simulink model "gfm_standalone"  (R2024a)
settings: Solver=VariableStepAuto  StartTime=0  StopTime=5  RelTol=1e-3
values from neighbouring files (symbols this model uses):
  Cf_pu = 0.03    [main__gfm.m]    (also in main_parallel.m; main_parallel_alt.m; main_standalone.m; scr.m)
  Cs_pu = 0.3    [main_parallel.m]    (also in main_parallel_alt.m; main_standalone.m)
  Dp = 0.02    [main__gfm.m]    (also in main_parallel.m; main_parallel_alt.m; main_standalone.m; scr.m)
  Dq = 0.3    [main__gfm.m]    (also in main_parallel.m; main_parallel_alt.m; main_standalone.m; scr.m)
  fac = 0    [main__gfm.m]    (also in main_parallel.m; main_parallel_alt.m; main_standalone.m; scr.m)
  H = 1.2    [main__gfm.m]    (also in main_parallel.m = 0.3; main_parallel_alt.m = 0.3; main_standalone.m; scr.m)
  I_load = Vpcc0/Zload_pu    [main__gfm.m]    (also in main_parallel.m = Vpcc/Zload_pu; main_parallel_alt.m = Vpoc/Zload_pu; main_standalone.m; scr.m)
  Ic = (Vconv-Vlcl)/(Rc_pu+1i*Lc_pu)    [main__gfm.m]    (also in main_standalone.m; scr.m; ss_RX.m; test_droop_gain.m)
  If = (Vlcl - Vload) / Zf_pu    [main_standalone.m]
  Ig = (Vlcl - Vinf) / Z_pu    [main__gfm.m]    (also in main_standalone.m = (Vload - Vinf) / Z_pu; scr.m; ss_RX.m; test_droop_gain.m)
  kfi = 0    [main__gfm.m]    (also in main_parallel.m; main_parallel_alt.m; main_standalone.m; scr.m)
  kii = Rc_pu / L * kpi    [main__gfm.m]    (also in main_parallel.m; main_parallel_alt.m; main_standalone.m; scr.m)
  kiq = 0.1    [main__gfm.m]    (also in main_parallel.m = 0.01; main_parallel_alt.m = 0.01; main_standalone.m; scr.m)
  kivd = 100    [main__gfm.m]    (also in main_parallel.m = 50; main_parallel_alt.m = 50; main_standalone.m; scr.m)
  kivq = 100    [main__gfm.m]    (also in main_parallel.m = 50; main_parallel_alt.m = 50; main_standalone.m; scr.m)
  kpi = 2 * pi * f_bw * L    [main__gfm.m]    (also in main_parallel.m; main_parallel_alt.m; main_standalone.m; scr.m)
  kpvd = 0.1    [main__gfm.m]    (also in main_parallel.m = 0.45; main_parallel_alt.m = 0.45; main_standalone.m; scr.m)
  kpvq = 0.1    [main__gfm.m]    (also in main_parallel.m = 0.45; main_parallel_alt.m = 0.45; main_standalone.m; scr.m = 1)
  Lc_pu = Lc / Lb    [main__gfm.m]    (also in main_parallel.m; main_parallel_alt.m; main_standalone.m; scr.m)
  Lg_pu = 0.5    [main__gfm.m]    (also in main_parallel.m = 0.0166666666667; main_parallel_alt.m = 0.0166666666667; main_standalone.m; scr.m = Lg_pux)
  Lgf_pu = Lgf/Lb    (= 0.0166666666667)    [main_parallel.m]    (also in main_parallel_alt.m; main_standalone.m)
  mu = 0.005    [main__gfm.m]    (also in main_standalone.m; scr.m; ss_RX.m; test_droop_gain.m)
  Pref = -line_flow(3,4)    [main__gfm.m]    (also in main_standalone.m = -line_flow(5,4); scr.m; ss_RX.m; test_droop_gain.m)
  PsiId0 = real(Vconv_c)-real(Vpcc_c)+X*imag(Ipcc_c)    [main__gfm.m]    (also in main_standalone.m; scr.m; ss_RX.m; test_droop_gain.m)
  PsiIq0 = imag(Vconv_c)-imag(Vpcc_c)-X*real(Ipcc_c)    [main__gfm.m]    (also in main_standalone.m; scr.m; ss_RX.m; test_droop_gain.m)
  PsiP0 = real(Ipcc_c)-wCpu*imag(Vpcc_c)*fac+imag(Ipcc_c)*kfi    [main__gfm.m]    (also in main_standalone.m; scr.m; ss_RX.m; test_droop_gain.m)
  PsiV0 = imag(Ipcc_c)+wCpu*real(Vpcc_c)*fac+real(Ipcc_c)*kfi    [main__gfm.m]    (also in main_standalone.m; scr.m; ss_RX.m; test_droop_gain.m)
  Qref = -line_flow(3,5)    [main__gfm.m]    (also in main_standalone.m = -line_flow(5,5); scr.m; ss_RX.m; test_droop_gain.m)
  Rc_pu = Rc / Zb    (= 5.19390581717e-06)    [main__gfm.m]    (also in main_parallel.m; main_parallel_alt.m; main_standalone.m; scr.m)
  Rf_pu = Rf / Zb    [main__gfm.m]    (also in main_parallel.m; main_parallel_alt.m; main_standalone.m; scr.m)
  Rg_pu = XrXg*Lg_pu    (= 0)    [main__gfm.m]    (also in main_standalone.m; scr.m; ss_RX.m; test_droop_gain.m)
  Rs_pu = 0.1    [main_parallel.m]    (also in main_parallel_alt.m; main_standalone.m)
  Vcf0 = Vlcl+Rf_pu*Icf    [main__gfm.m]    (also in main_standalone.m; scr.m; ss_RX.m; test_droop_gain.m)
  Vconv_c = Vconv * exp(-1i*theta_ref)    [main__gfm.m]    (also in main_standalone.m; scr.m; ss_RX.m; test_droop_gain.m)
  Vinf = V0(3,1)    [main__gfm.m]    (also in main_parallel.m = V0(6,1); main_parallel_alt.m = V0(6,1); main_standalone.m = V0(4,1); scr.m)
  Vpcc0 = Vlcl    [main__gfm.m]    (also in main_standalone.m = Vload; scr.m; ss_RX.m; test_droop_gain.m)
  Vs = Vpcc + Rs_pu*Igf    [main_parallel.m]    (also in main_parallel_alt.m = Vpoc + Rs_pu*Igf; main_standalone.m = Vload+Rs_pu*Ibf)
  wCpu = Zb * wb * Cf    (= 0.03)    [main__gfm.m]    (also in main_parallel.m; main_parallel_alt.m; main_standalone.m; scr.m)
  wLpu = X    [main__gfm.m]    (also in main_parallel.m; main_parallel_alt.m; main_standalone.m; scr.m)
  Zload_pu = inv(YL(2,2))    [main__gfm.m]    (also in main_parallel.m = inv(YL(3,3)); main_parallel_alt.m = inv(YL(3,3)); main_standalone.m = inv(YL(3,3)); scr.m)
settings Model: Creator=HP  LastModifiedBy=HP
settings DataIOCC: SaveFormat=StructureWithTime
settings OptimizationCC: BlockReduction=off  BufferReuse=off
settings DebuggingCC: AlgebraicLoopMsg=none

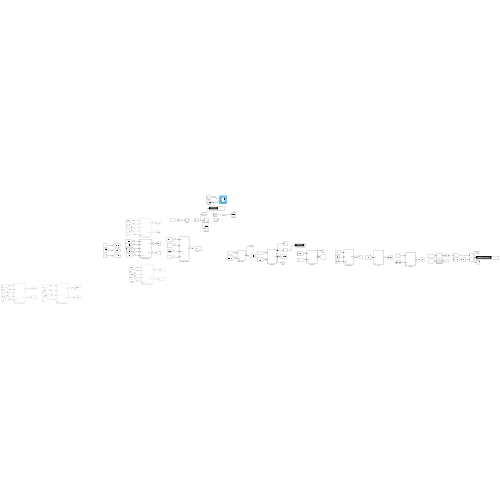
[thumbnail: Simulink's stored preview of the top-level diagram]
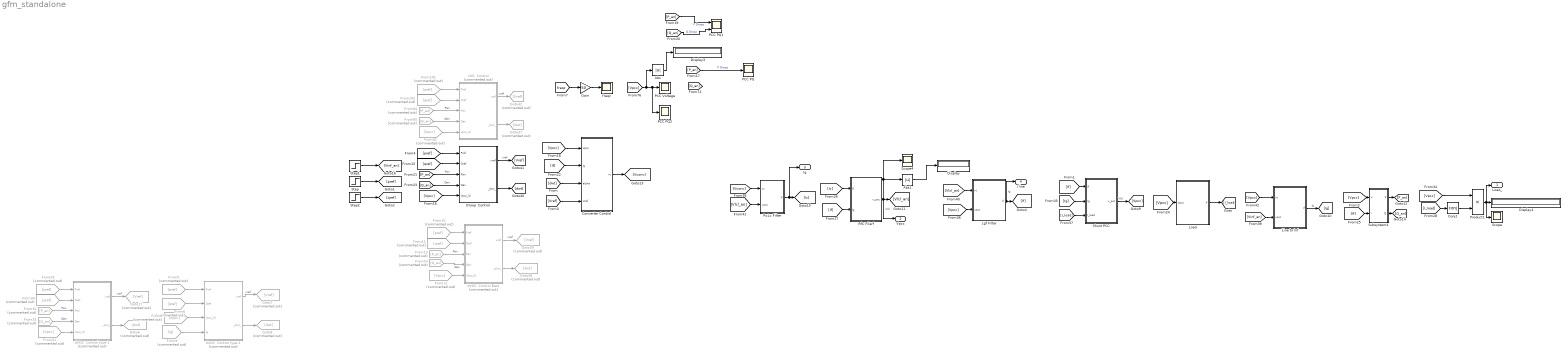
== system gfm_standalone ==
  Abs : Abs  SaturateOnIntegerOverflow=off
  Abs1 : Abs  SaturateOnIntegerOverflow=off
  Conj2 : Math  Operator=conj
  Converter Control : Subsystem
  Display : Display
  Display3 : Display
  Display4 : Display
  Droop  Control : Subsystem  mask{md=Dp, nd=Dq, kiq=0, vref_=Vpcc0}
      mask prompts: md "P droop gain"; nd "Q droop gain"; kiq "KiQ-V"; vref_ "Voltage ref"
      mask DialogControl DescGroupVar Prompt: Outer Control
      mask DialogControl DescTextVar Prompt: Droop Control Block by HIP
  From{5,10,29,101} (4 alike) : From  Commented=on  GotoTag=pref
  From{6,11,30,102} (4 alike) : From  Commented=on  GotoTag=qref
  From{8,12,31,92} (4 alike) : From  Commented=on  GotoTag=Vpcc
  From13 : From  Commented=on  GotoTag=P_an
  From14 : From  Commented=on  GotoTag=Q_an
  From32 : From  Commented=on  GotoTag=P_an
  From33 : From  Commented=on  GotoTag=Q_an
  From9 : From  Commented=on  GotoTag=Ig
  From94 : From  Commented=on  GotoTag=P_an
  From95 : From  Commented=on  GotoTag=Q_an
  Gain : Gain  Gain=50
  Goto{7,17,39,42} (4 alike) : Goto  Commented=on  GotoTag=Vref
  Goto{6,8,37..38} (4 alike) : Goto  Commented=on  GotoTag=dwt
  Lgf Filter : Subsystem  mask{i0=If, R=0, L=Lgf_pu}
      mask prompts: i0 "I initial condition (pu)"; R "R (pu)"; L "L (pu)"
  Line to Inf : Subsystem  mask{i0=Ig, R=Rg_pu, L=Lg_pu}
      mask prompts: i0 "I initial condition (pu)"; R "R (pu)"; L "L (pu)"
  Load : Subsystem  mask{i0=I_load, R=real(Zload_pu), L=imag(Zload_pu)}
      mask prompts: i0 "I initial condition (pu)"; R "R (pu)"; L "L (pu)"
  PCC PQ : Scope
  PCC PQ1 : Scope  NumInputPorts=2
  PCC PQ2 : Scope
  PCC Voltage : Scope
  Product1 : Product
  RcLc Filter : Subsystem  mask{i0=Ic, R=Rc_pu, L=Lc_pu}
      mask prompts: i0 "I initial condition (pu)"; R "R (pu)"; L "L (pu)"
  RfC Filerf : Subsystem  mask{vc0=Vcf0, R=Rf_pu, C=Cf_pu}
      mask prompts: vc0 "initial value Vpcc  (p.u.)"; R "R (pu)"; C "C (pu)"
  Scope : Scope
  Scope4 : Scope
  Shunt PCC : Subsystem  mask{vc0=Vs, R=Rs_pu, C=Cs_pu}
      mask prompts: vc0 "initial value Vpcc  (p.u.)"; R "R (pu)"; C "C (pu)"
  Step : Step  Before=Pref  SampleTime=0
  Step1 : Step  Time=2  Before=Vinf  After=Vinf  SampleTime=0
  Step2 : Step  Before=Qref  After=0.2  SampleTime=0
  Subsystem4 : Subsystem
  VSG  Control : Subsystem  Commented=on  mask{Dp=50, H=H, nd=Dq, kiq=kiq, vref_=Vpcc0}
      mask prompts: Dp "Dp (damping factor)"; H "Inertia Constant"; nd "VSG Q gain"; kiq "KiQ-V"; vref_ "Voltage ref"
      mask DialogControl DescGroupVar Prompt: Outer Control
      mask DialogControl DescTextVar Prompt: VSG Control Block by HIP
  dVOC  Control Best : Subsystem  Commented=on  mask{md=Dp, nd=Dq, mu=mu, vref_=Vpcc0}
      mask prompts: md "P droop gain"; nd "Q droop gain"; mu "mu (V)"; vref_ "Voltage ref"
      mask DialogControl DescGroupVar Prompt: Outer Control
      mask DialogControl DescTextVar Prompt: dVOC Control Block by HIP
  dVOC  Control type 1 : Subsystem  Commented=on  mask{md=Dp, nd=Dq, mu=mu, vref_=Vpcc0}
      mask prompts: md "P droop gain"; nd "Q droop gain"; mu "mu (V)"; vref_ "Voltage ref"
      mask DialogControl DescGroupVar Prompt: Outer Control
      mask DialogControl DescTextVar Prompt: dVOC Control Block by HIP
  dVOC  Control type 2 : Subsystem  Commented=on  mask{md=Dp, nd=Dq, mu=mu, vref_=Vpcc0}
      mask prompts: md "P droop gain"; nd "Q droop gain"; mu "mu (V)"; vref_ "Voltage ref"
      mask DialogControl DescGroupVar Prompt: Outer Control
      mask DialogControl DescTextVar Prompt: dVOC Control Block by HIP
  freqz : Scope
  Load_ : Outport
  Vpcc : Outport  Port=2
  Ig : Outport  Port=3
  I line : Outport  Port=4
  wires:
  [If] -> Converter Control/2(Ig)
  [Vref] -> Converter Control/4(Vref)
  [Vpcc] -> Converter Control/1(Vpcc)
  Converter Control/1(vt) -> [Vconv]
  [dwt] -> Converter Control/3(alpha)
  Step/1 -> [pref]
  Step1/1 -> [Vinf_an]
  Step2/1 -> [qref]
  Gain/1 -> freqz/1
  [freqz] -> Gain/1
  [Vpcc] -> Abs/1, PCC PQ2/1, PCC Voltage/1
  Droop  Control/1(vref) -> [Vref]  "vref"
  From92/1 -> VSG  Control/5(Vpcc_lcl)
  From95/1 -> VSG  Control/4(Qan)  "Qan"
  VSG  Control/2(_dwt_) -> Goto37/1
  Droop  Control/2(_dwt_) -> [dwt]
  From102/1 -> VSG  Control/2(Qref)
  From101/1 -> VSG  Control/1(Pref)
  From94/1 -> VSG  Control/3(Pan)  "Pan"
  VSG  Control/1(vref) -> Goto42/1  "vref"
  [pref] -> Droop  Control/1(Pref)
  [qref] -> Droop  Control/2(Qref)
  [Q_an] -> Droop  Control/4(Qan)  "Qan"
  [P_an] -> Droop  Control/3(Pan)  "Pan"
  [Vpcc] -> Droop  Control/5(Vpcc_lcl)
  [P_an] -> PCC PQ/1  "P Droop"
  dVOC  Control type 1/1(vref) -> Goto17/1  "vref"
  From30/1 -> dVOC  Control type 1/2(Qref)
  dVOC  Control type 1/2(_dwt_) -> Goto6/1
  From29/1 -> dVOC  Control type 1/1(Pref)
  From33/1 -> dVOC  Control type 1/4(Qan)  "Qan"
  From32/1 -> dVOC  Control type 1/3(Pan)  "Pan"
  From31/1 -> dVOC  Control type 1/5(Vpcc_lcl)
  From8/1 -> dVOC  Control type 2/3(Vpcc_lcl)
  From5/1 -> dVOC  Control type 2/1(Pref)
  From6/1 -> dVOC  Control type 2/2(Qref)
  dVOC  Control type 2/2(_dwt_) -> Goto8/1
  dVOC  Control type 2/1(vref) -> Goto7/1  "vref"
  From9/1 -> dVOC  Control type 2/4(Ig)
  Abs/1 -> Display3/1
  dVOC  Control Best/1(vref) -> Goto39/1  "vref"
  dVOC  Control Best/2(_dwt_) -> Goto38/1
  From10/1 -> dVOC  Control Best/1(Pref)
  From11/1 -> dVOC  Control Best/2(Qref)
  From13/1 -> dVOC  Control Best/3(Pan)  "Pan"
  From14/1 -> dVOC  Control Best/4(Qan)  "Qan"
  From12/1 -> dVOC  Control Best/5(Vpcc_lcl)
  [Q_an] -> PCC PQ1/2  "Q Droop"
  [P_an] -> PCC PQ1/1  "P Droop"
  [Vinf_an] -> Line to Inf/2("vpcc ")
  [If] -> RfC Filerf/2("Ig ")
  RcLc Filter/1(if) -> Ig/1, [Ic]
  [Vconv] -> RcLc Filter/1("vt ")
  Lgf Filter/1(if) -> I line/1, [If]  "Ig"
  [Vpcc] -> Subsystem4/1(V)
  [Vpcc] -> Line to Inf/1("vt ")
  [Vlcl_an] -> Lgf Filter/1("vt ")
  [If] -> Subsystem4/2(I)
  Conj2/1 -> Product1/2
  RfC Filerf/1(v_pcc) -> Vpcc/1, Abs1/1, Scope4/1, [Vlcl_an]  "Vlcl"
  Product1/1 -> Load_/1, Scope/1, Display4/1
  [Ic] -> RfC Filerf/1("If ")
  Line to Inf/1(if) -> [Ig]  "Ig"
  [If] -> Shunt PCC/1("If ")
  [I_load] -> Shunt PCC/3(I_load)
  [I_load] -> Conj2/1
  [Ig] -> Shunt PCC/2("Ig ")
  Subsystem4/1(P) -> [P_an]
  [Vpcc] -> Load/1("Vpcc ")
  [Vpcc] -> Lgf Filter/2("vpcc ")
  [Vlcl_an] -> RcLc Filter/2("vpcc ")
  [Vpcc] -> Product1/1
  Abs1/1 -> Display/1
  Subsystem4/2(Q) -> [Q_an]
  Load/1(if) -> [I_load]
  Shunt PCC/1(v_pcc) -> [Vpcc]  "Vlcl"

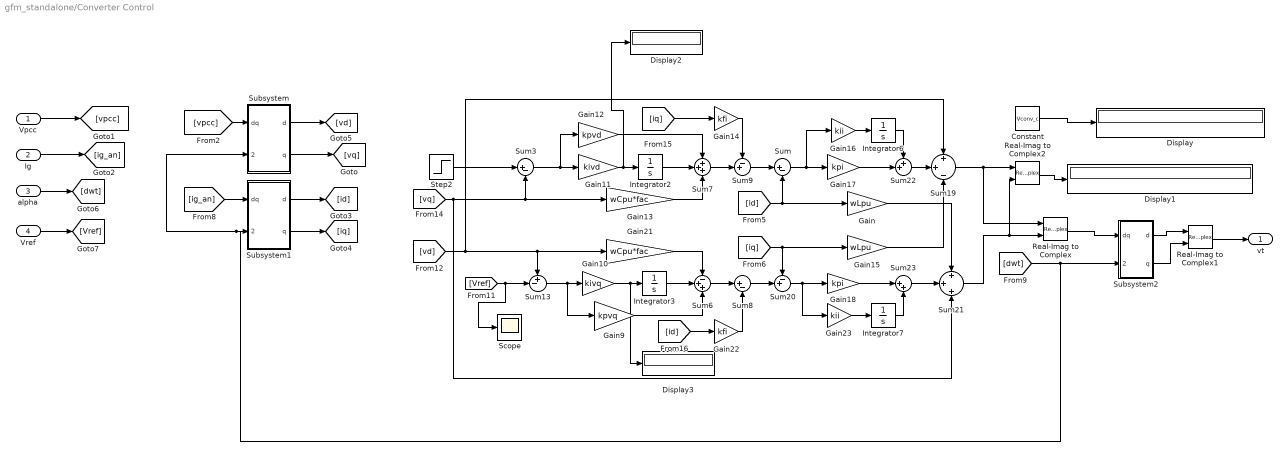
== system gfm_standalone/Converter Control ==
  Vpcc : Inport
  Ig : Inport  Port=2
  alpha : Inport  Port=3
  Vref : Inport  Port=4
  Constant : Constant  Value=Vconv_c
  Display{,1..3} (4 alike) : Display
  Gain : Gain  Gain=wLpu
  Gain10 : Gain  Gain=kivq
  Gain11 : Gain  Gain=kivd
  Gain12 : Gain  Gain=kpvd
  Gain13 : Gain  Gain=wCpu*fac
  Gain14 : Gain  Gain=kfi
  Gain15 : Gain  Gain=wLpu
  Gain16 : Gain  Gain=kii
  Gain17 : Gain  Gain=kpi
  Gain18 : Gain  Gain=kpi
  Gain21 : Gain  Gain=wCpu*fac
  Gain22 : Gain  Gain=kfi
  Gain23 : Gain  Gain=kii
  Gain9 : Gain  Gain=kpvq
  Integrator2 : Integrator  InitialCondition=PsiP0  ContinuousStateAttributes='psi_alpha'
  Integrator3 : Integrator  InitialCondition=PsiV0  ContinuousStateAttributes='psiV'
  Integrator6 : Integrator  InitialCondition=PsiId0  ContinuousStateAttributes='psi_id'
  Integrator7 : Integrator  InitialCondition=PsiIq0  ContinuousStateAttributes='psi_iq'
  Real-Imag to Complex : RealImagToComplex
  Real-Imag to Complex1 : RealImagToComplex
  Real-Imag to Complex2 : RealImagToComplex
  Scope : Scope
  Step2 : Step  After=0  SampleTime=0
  Subsystem : Subsystem
  Subsystem1 : Subsystem
  Subsystem2 : Subsystem
  Sum : Sum  Inputs=|+-
  Sum13 : Sum  Inputs=+-|
  Sum19 : Sum  Inputs=+|+|-
  Sum20 : Sum  Inputs=-+|
  Sum21 : Sum  Inputs=+|+|+
  Sum22 : Sum  Inputs=++|
  Sum23 : Sum  Inputs=|++
  Sum3 : Sum  Inputs=|+-
  Sum6 : Sum  Inputs=-++
  Sum7 : Sum  Inputs=+++
  Sum8 : Sum  Inputs=|+-
  Sum9 : Sum  Inputs=-+|
  vt : Outport
  wires:
  Integrator3/1 -> Sum6/2
  Gain11/1 -> Display2/1, Integrator2/1
  Subsystem/2(q) -> [vq]
  Sum13/1 -> Gain10/1, Gain9/1
  Ig/1 -> [ig_an]
  [vpcc] -> Subsystem/1(dq)
  Subsystem2/2(q) -> Real-Imag to Complex1/2
  Subsystem2/1(d) -> Real-Imag to Complex1/1
  Real-Imag to Complex/1 -> Subsystem2/1(dq)
  [id] -> Sum/2, Gain/1
  Subsystem1/1(d) -> [id]
  [iq] -> Gain15/1, Sum20/1
  Sum21/1 -> Real-Imag to Complex2/2, Real-Imag to Complex/2
  Integrator6/1 -> Sum22/1
  Sum20/1 -> Gain23/1, Gain18/1
  Gain23/1 -> Integrator7/1
  Gain18/1 -> Sum23/1
  Sum22/1 -> Sum19/2
  Gain22/1 -> Sum8/2
  Gain10/1 -> Display3/1, Integrator3/1
  Gain14/1 -> Sum9/1
  Sum8/1 -> Sum20/2
  Sum7/1 -> Sum9/2
  [ig_an] -> Subsystem1/1(dq)
  Gain13/1 -> Sum7/3
  Sum19/1 -> Real-Imag to Complex/1, Real-Imag to Complex2/1
  Sum3/1 -> Gain12/1, Gain11/1
  Gain16/1 -> Integrator6/1
  Sum/1 -> Gain16/1, Gain17/1
  Gain/1 -> Sum21/1
  [Vref] -> Scope/1, Sum13/2
  Gain9/1 -> Sum6/3
  Gain21/1 -> Sum6/1
  Subsystem1/2(q) -> [iq]
  Integrator7/1 -> Sum23/2
  Sum23/1 -> Sum21/2
  Subsystem/1(d) -> [vd]
  [vq] -> Sum3/2, Gain13/1, Sum21/3
  Gain15/1 -> Sum19/3
  [vd] -> Gain21/1, Sum13/1, Sum19/1
  Gain17/1 -> Sum22/2
  [id] -> Gain22/1
  [iq] -> Gain14/1
  Vpcc/1 -> [vpcc]
  Gain12/1 -> Sum7/1
  Sum6/1 -> Sum8/1
  Integrator2/1 -> Sum7/2
  Real-Imag to Complex1/1 -> vt/1
  Sum9/1 -> Sum/1
  [dwt] -> Subsystem1/2(delta_wt), Subsystem/2(delta_wt), Subsystem2/2(d_wt)
  Step2/1 -> Sum3/1
  alpha/1 -> [dwt]
  Vref/1 -> [Vref]
  Constant/1 -> Display/1
  Real-Imag to Complex2/1 -> Display1/1

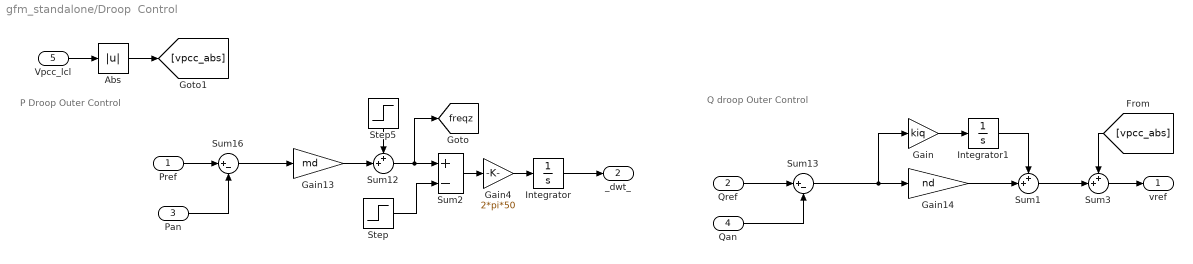
== system gfm_standalone/Droop  Control ==
  note: Q droop Outer Control
  note: P Droop Outer Control
  Pref : Inport
  Qref : Inport  Port=2
  Pan : Inport  Port=3
  Qan : Inport  Port=4
  Vpcc_lcl : Inport  Port=5
  Abs : Abs  SaturateOnIntegerOverflow=off
  Gain : Gain  Gain=kiq
  Gain13 : Gain  Gain=md
  Gain14 : Gain  Gain=nd
  Gain4 : Gain  Gain=2*pi*50
  Integrator : Integrator  InitialCondition=angle(vref_)  ContinuousStateAttributes='theta0'
  Integrator1 : Integrator
  Step : Step  Before=1.00  After=1.000  SampleTime=0
  Step5 : Step  Time=2  Before=1  SampleTime=0
  Sum1 : Sum  Inputs=++|
  Sum12 : Sum  Inputs=++|
  Sum13 : Sum  Inputs=|+-
  Sum16 : Sum  Inputs=|+-
  Sum2 : Sum  Inputs=+-
  Sum3 : Sum  Inputs=++|
  vref : Outport
  _dwt_ : Outport  Port=2
  tag scope: freqz=global
  wires:
  Gain13/1 -> Sum12/2
  Qref/1 -> Sum13/1
  Sum3/1 -> vref/1
  Qan/1 -> Sum13/2
  Pref/1 -> Sum16/1
  Pan/1 -> Sum16/2
  Sum13/1 -> Gain/1, Gain14/1
  Sum2/1 -> Gain4/1
  Gain4/1 -> Integrator/1
  Sum12/1 -> Sum2/1, [freqz]
  Integrator/1 -> _dwt_/1
  Sum16/1 -> Gain13/1
  Step5/1 -> Sum12/1
  Step/1 -> Sum2/2
  Gain/1 -> Integrator1/1
  Gain14/1 -> Sum1/2
  Integrator1/1 -> Sum1/1
  Sum1/1 -> Sum3/2
  Vpcc_lcl/1 -> Abs/1
  Abs/1 -> [vpcc_abs]
  [vpcc_abs] -> Sum3/1

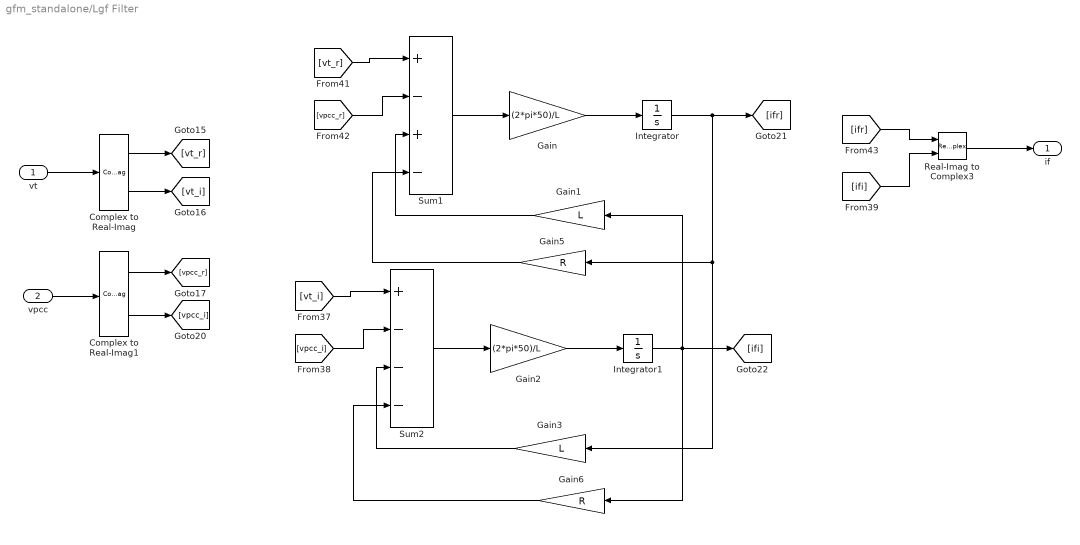
== system gfm_standalone/Lgf Filter ==
  "vt " : Inport
  "vpcc " : Inport  Port=2
  Complex to Real-Imag : ComplexToRealImag
  Complex to Real-Imag1 : ComplexToRealImag
  Gain : Gain  Gain=(2*pi*50)/L
  Gain1 : Gain  Gain=L
  Gain2 : Gain  Gain=(2*pi*50)/L
  Gain3 : Gain  Gain=L
  Gain5 : Gain  Gain=R
  Gain6 : Gain  Gain=R
  Integrator : Integrator  InitialCondition=real(i0)  ContinuousStateAttributes='iline1_re'
  Integrator1 : Integrator  InitialCondition=imag(i0)  ContinuousStateAttributes='iline1_im'
  Real-Imag to Complex3 : RealImagToComplex
  Sum1 : Sum  Inputs=+-+-
  Sum2 : Sum  Inputs=+---
  if : Outport
  wires:
  "vpcc "/1 -> Complex to Real-Imag1/1
  Gain5/1 -> Sum1/4
  Real-Imag to Complex3/1 -> if/1
  Integrator1/1 -> Gain6/1, Gain1/1, [ifi]
  [ifr] -> Real-Imag to Complex3/1
  "vt "/1 -> Complex to Real-Imag/1
  Integrator/1 -> Gain5/1, Gain3/1, [ifr]
  [ifi] -> Real-Imag to Complex3/2
  [vpcc_r] -> Sum1/2
  Gain6/1 -> Sum2/4
  Complex to Real-Imag/1 -> [vt_r]
  Gain1/1 -> Sum1/3
  Complex to Real-Imag/2 -> [vt_i]
  Complex to Real-Imag1/1 -> [vpcc_r]
  Sum2/1 -> Gain2/1
  Gain2/1 -> Integrator1/1
  [vt_i] -> Sum2/1
  [vpcc_i] -> Sum2/2
  [vt_r] -> Sum1/1
  Gain3/1 -> Sum2/3
  Complex to Real-Imag1/2 -> [vpcc_i]
  Gain/1 -> Integrator/1
  Sum1/1 -> Gain/1

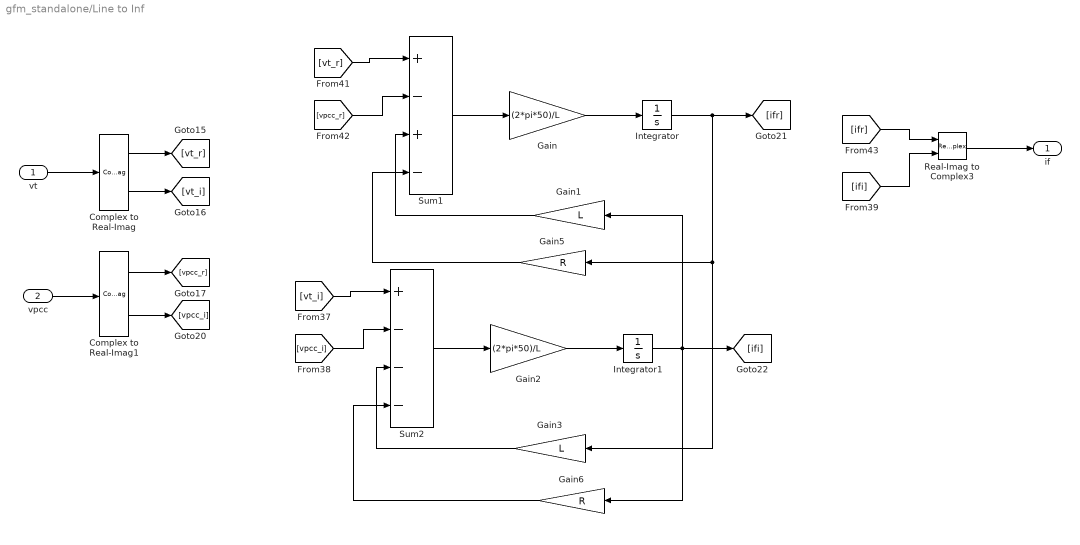
== system gfm_standalone/Line to Inf ==
  "vt " : Inport
  "vpcc " : Inport  Port=2
  Complex to Real-Imag : ComplexToRealImag
  Complex to Real-Imag1 : ComplexToRealImag
  Gain : Gain  Gain=(2*pi*50)/L
  Gain1 : Gain  Gain=L
  Gain2 : Gain  Gain=(2*pi*50)/L
  Gain3 : Gain  Gain=L
  Gain5 : Gain  Gain=R
  Gain6 : Gain  Gain=R
  Integrator : Integrator  InitialCondition=real(i0)  ContinuousStateAttributes='iline1_re'
  Integrator1 : Integrator  InitialCondition=imag(i0)  ContinuousStateAttributes='iline1_im'
  Real-Imag to Complex3 : RealImagToComplex
  Sum1 : Sum  Inputs=+-+-
  Sum2 : Sum  Inputs=+---
  if : Outport
  wires:
  "vpcc "/1 -> Complex to Real-Imag1/1
  Gain5/1 -> Sum1/4
  Real-Imag to Complex3/1 -> if/1
  Integrator1/1 -> Gain6/1, Gain1/1, [ifi]
  [ifr] -> Real-Imag to Complex3/1
  "vt "/1 -> Complex to Real-Imag/1
  Integrator/1 -> Gain5/1, Gain3/1, [ifr]
  [ifi] -> Real-Imag to Complex3/2
  [vpcc_r] -> Sum1/2
  Gain6/1 -> Sum2/4
  Complex to Real-Imag/1 -> [vt_r]
  Gain1/1 -> Sum1/3
  Complex to Real-Imag/2 -> [vt_i]
  Complex to Real-Imag1/1 -> [vpcc_r]
  Sum2/1 -> Gain2/1
  Gain2/1 -> Integrator1/1
  [vt_i] -> Sum2/1
  [vpcc_i] -> Sum2/2
  [vt_r] -> Sum1/1
  Gain3/1 -> Sum2/3
  Complex to Real-Imag1/2 -> [vpcc_i]
  Gain/1 -> Integrator/1
  Sum1/1 -> Gain/1

== system gfm_standalone/Load ==
  "Vpcc " : Inport
  Complex to Real-Imag : ComplexToRealImag
  Gain : Gain  Gain=(2*pi*50)/L
  Gain1 : Gain  Gain=L
  Gain2 : Gain  Gain=(2*pi*50)/L
  Gain3 : Gain  Gain=L
  Gain5 : Gain  Gain=R
  Gain6 : Gain  Gain=R
  Integrator : Integrator  InitialCondition=real(i0)  ContinuousStateAttributes='iload_re'
  Integrator1 : Integrator  InitialCondition=imag(i0)  ContinuousStateAttributes='iload_im'
  Real-Imag to Complex3 : RealImagToComplex
  Sum1 : Sum  Inputs=+-+-
  Sum2 : Sum  Inputs=+---
  if : Outport
  wires:
  Gain5/1 -> Sum1/4
  Real-Imag to Complex3/1 -> if/1
  Integrator1/1 -> Gain6/1, Gain1/1, [ifi]
  [ifr] -> Real-Imag to Complex3/1
  "Vpcc "/1 -> Complex to Real-Imag/1
  Integrator/1 -> Gain5/1, Gain3/1, [ifr]
  [ifi] -> Real-Imag to Complex3/2
  Gain6/1 -> Sum2/4
  Complex to Real-Imag/1 -> [vt_r]
  Gain1/1 -> Sum1/3
  Complex to Real-Imag/2 -> [vt_i]
  Sum2/1 -> Gain2/1
  Gain2/1 -> Integrator1/1
  [vt_i] -> Sum2/1
  [vt_r] -> Sum1/1
  Gain3/1 -> Sum2/3
  Gain/1 -> Integrator/1
  Sum1/1 -> Gain/1

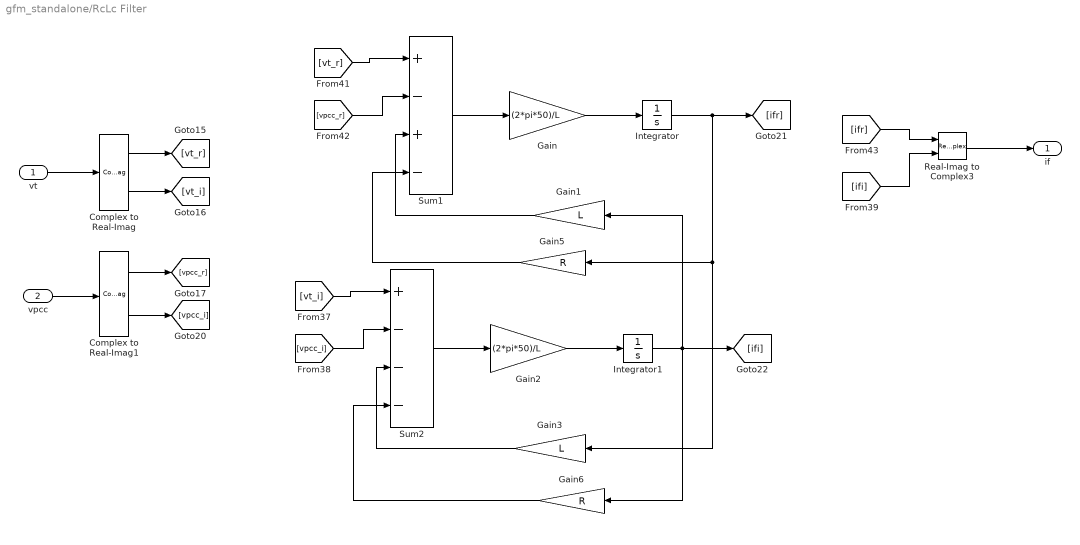
== system gfm_standalone/RcLc Filter ==
  "vt " : Inport
  "vpcc " : Inport  Port=2
  Complex to Real-Imag : ComplexToRealImag
  Complex to Real-Imag1 : ComplexToRealImag
  Gain : Gain  Gain=(2*pi*50)/L
  Gain1 : Gain  Gain=L
  Gain2 : Gain  Gain=(2*pi*50)/L
  Gain3 : Gain  Gain=L
  Gain5 : Gain  Gain=R
  Gain6 : Gain  Gain=R
  Integrator : Integrator  InitialCondition=real(i0)  ContinuousStateAttributes='ig_re'
  Integrator1 : Integrator  InitialCondition=imag(i0)  ContinuousStateAttributes='ig_im'
  Real-Imag to Complex3 : RealImagToComplex
  Sum1 : Sum  Inputs=+-+-
  Sum2 : Sum  Inputs=+---
  if : Outport
  wires:
  "vpcc "/1 -> Complex to Real-Imag1/1
  Gain5/1 -> Sum1/4
  Real-Imag to Complex3/1 -> if/1
  Integrator1/1 -> Gain6/1, Gain1/1, [ifi]
  [ifr] -> Real-Imag to Complex3/1
  "vt "/1 -> Complex to Real-Imag/1
  Integrator/1 -> Gain5/1, Gain3/1, [ifr]
  [ifi] -> Real-Imag to Complex3/2
  [vpcc_r] -> Sum1/2
  Gain6/1 -> Sum2/4
  Complex to Real-Imag/1 -> [vt_r]
  Gain1/1 -> Sum1/3
  Complex to Real-Imag/2 -> [vt_i]
  Complex to Real-Imag1/1 -> [vpcc_r]
  Sum2/1 -> Gain2/1
  Gain2/1 -> Integrator1/1
  [vt_i] -> Sum2/1
  [vpcc_i] -> Sum2/2
  [vt_r] -> Sum1/1
  Gain3/1 -> Sum2/3
  Complex to Real-Imag1/2 -> [vpcc_i]
  Gain/1 -> Integrator/1
  Sum1/1 -> Gain/1

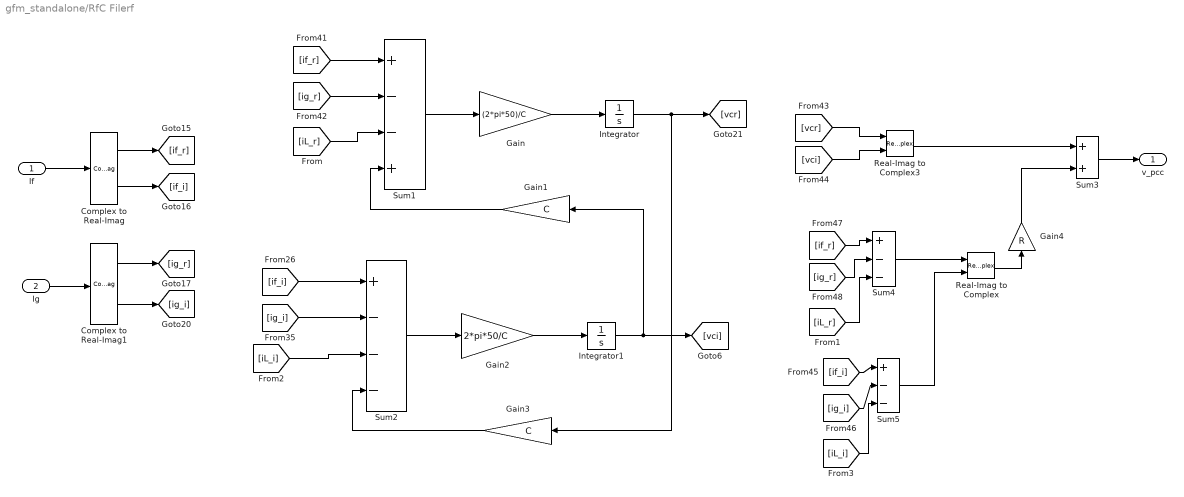
== system gfm_standalone/RfC Filerf ==
  "If " : Inport
  "Ig " : Inport  Port=2
  Complex to Real-Imag : ComplexToRealImag
  Complex to Real-Imag1 : ComplexToRealImag
  Gain : Gain  Gain=(2*pi*50)/C
  Gain1 : Gain  Gain=C
  Gain2 : Gain  Gain=2*pi*50/C
  Gain3 : Gain  Gain=C
  Gain4 : Gain  Gain=R
  Integrator : Integrator  InitialCondition=real(vc0)  ContinuousStateAttributes='vpcc_re'
  Integrator1 : Integrator  InitialCondition=imag(vc0)  ContinuousStateAttributes='vpcc_im'
  Real-Imag to Complex : RealImagToComplex
  Real-Imag to Complex3 : RealImagToComplex
  Sum1 : Sum  Inputs=+--+
  Sum2 : Sum  Inputs=+---
  Sum3 : Sum
  Sum4 : Sum  Inputs=+--
  Sum5 : Sum  Inputs=+--
  v_pcc : Outport
  wires:
  Sum4/1 -> Real-Imag to Complex/1
  "Ig "/1 -> Complex to Real-Imag1/1
  Complex to Real-Imag1/2 -> [ig_i]
  Integrator1/1 -> Gain1/1, [vci]
  Sum1/1 -> Gain/1
  Gain/1 -> Integrator/1
  [ig_r] -> Sum1/2
  Real-Imag to Complex/1 -> Gain4/1
  [ig_r] -> Sum4/2
  [ig_i] -> Sum5/2
  Integrator/1 -> Gain3/1, [vcr]
  [ig_i] -> Sum2/2
  Gain2/1 -> Integrator1/1
  "If "/1 -> Complex to Real-Imag/1
  [if_i] -> Sum2/1
  [if_r] -> Sum4/1
  Sum2/1 -> Gain2/1
  [if_r] -> Sum1/1
  Sum5/1 -> Real-Imag to Complex/2
  Sum3/1 -> v_pcc/1
  [if_i] -> Sum5/1
  Gain4/1 -> Sum3/2
  Complex to Real-Imag/2 -> [if_i]
  [vci] -> Real-Imag to Complex3/2
  Real-Imag to Complex3/1 -> Sum3/1
  Complex to Real-Imag1/1 -> [ig_r]
  Complex to Real-Imag/1 -> [if_r]
  [vcr] -> Real-Imag to Complex3/1
  Gain1/1 -> Sum1/4
  Gain3/1 -> Sum2/4
  [iL_r] -> Sum1/3
  [iL_r] -> Sum4/3
  [iL_i] -> Sum2/3
  [iL_i] -> Sum5/3

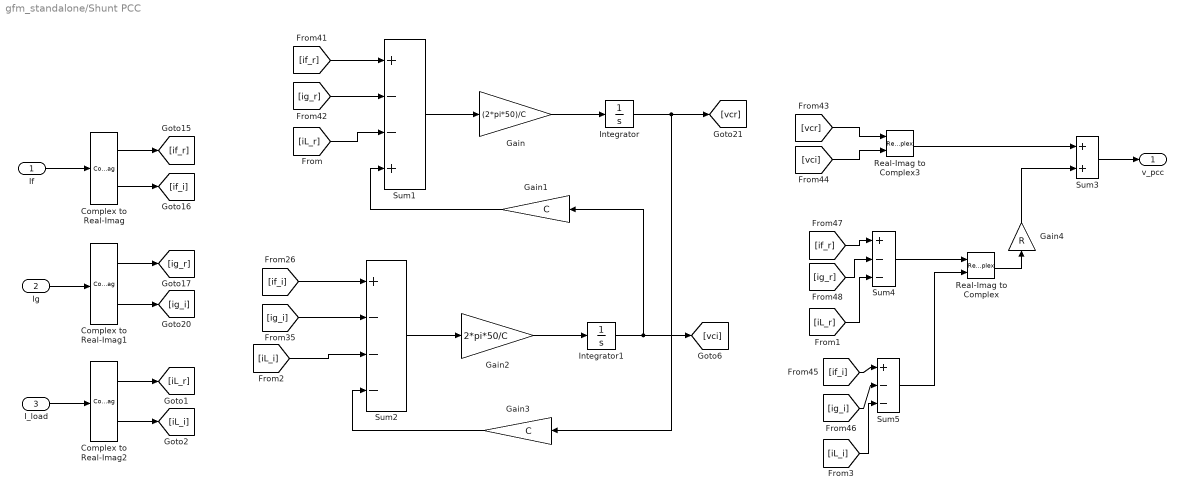
== system gfm_standalone/Shunt PCC ==
  "If " : Inport
  "Ig " : Inport  Port=2
  I_load : Inport  Port=3
  Complex to Real-Imag : ComplexToRealImag
  Complex to Real-Imag1 : ComplexToRealImag
  Complex to Real-Imag2 : ComplexToRealImag
  Gain : Gain  Gain=(2*pi*50)/C
  Gain1 : Gain  Gain=C
  Gain2 : Gain  Gain=2*pi*50/C
  Gain3 : Gain  Gain=C
  Gain4 : Gain  Gain=R
  Integrator : Integrator  InitialCondition=real(vc0)  ContinuousStateAttributes='vpcc_re'
  Integrator1 : Integrator  InitialCondition=imag(vc0)  ContinuousStateAttributes='vpcc_im'
  Real-Imag to Complex : RealImagToComplex
  Real-Imag to Complex3 : RealImagToComplex
  Sum1 : Sum  Inputs=+--+
  Sum2 : Sum  Inputs=+---
  Sum3 : Sum
  Sum4 : Sum  Inputs=+--
  Sum5 : Sum  Inputs=+--
  v_pcc : Outport
  wires:
  Sum4/1 -> Real-Imag to Complex/1
  "Ig "/1 -> Complex to Real-Imag1/1
  Complex to Real-Imag1/2 -> [ig_i]
  Integrator1/1 -> Gain1/1, [vci]
  Sum1/1 -> Gain/1
  Gain/1 -> Integrator/1
  [ig_r] -> Sum1/2
  Real-Imag to Complex/1 -> Gain4/1
  [ig_r] -> Sum4/2
  [ig_i] -> Sum5/2
  Integrator/1 -> Gain3/1, [vcr]
  [ig_i] -> Sum2/2
  Gain2/1 -> Integrator1/1
  "If "/1 -> Complex to Real-Imag/1
  [if_i] -> Sum2/1
  [if_r] -> Sum4/1
  Sum2/1 -> Gain2/1
  [if_r] -> Sum1/1
  Sum5/1 -> Real-Imag to Complex/2
  Sum3/1 -> v_pcc/1
  [if_i] -> Sum5/1
  Gain4/1 -> Sum3/2
  Complex to Real-Imag/2 -> [if_i]
  [vci] -> Real-Imag to Complex3/2
  Real-Imag to Complex3/1 -> Sum3/1
  Complex to Real-Imag1/1 -> [ig_r]
  Complex to Real-Imag/1 -> [if_r]
  [vcr] -> Real-Imag to Complex3/1
  Gain1/1 -> Sum1/4
  Gain3/1 -> Sum2/4
  Complex to Real-Imag2/1 -> [iL_r]
  Complex to Real-Imag2/2 -> [iL_i]
  I_load/1 -> Complex to Real-Imag2/1
  [iL_r] -> Sum1/3
  [iL_r] -> Sum4/3
  [iL_i] -> Sum2/3
  [iL_i] -> Sum5/3

== system gfm_standalone/Subsystem4 ==
  V : Inport
  I : Inport  Port=2
  Complex to Real-Imag : ComplexToRealImag
  Complex to Real-Imag1 : ComplexToRealImag
  Product{,1..3} (4 alike) : Product
  Sum : Sum
  Sum1 : Sum  Inputs=-+
  P : Outport
  Q : Outport  Port=2
  wires:
  Complex to Real-Imag/1 -> Product2/1, Product/1
  Sum1/1 -> Q/1
  V/1 -> Complex to Real-Imag/1
  Complex to Real-Imag1/2 -> Product2/2, Product1/2
  Product1/1 -> Sum/2
  Sum/1 -> P/1
  I/1 -> Complex to Real-Imag1/1
  Complex to Real-Imag/2 -> Product3/1, Product1/1
  Complex to Real-Imag1/1 -> Product/2, Product3/2
  Product/1 -> Sum/1
  Product3/1 -> Sum1/2
  Product2/1 -> Sum1/1

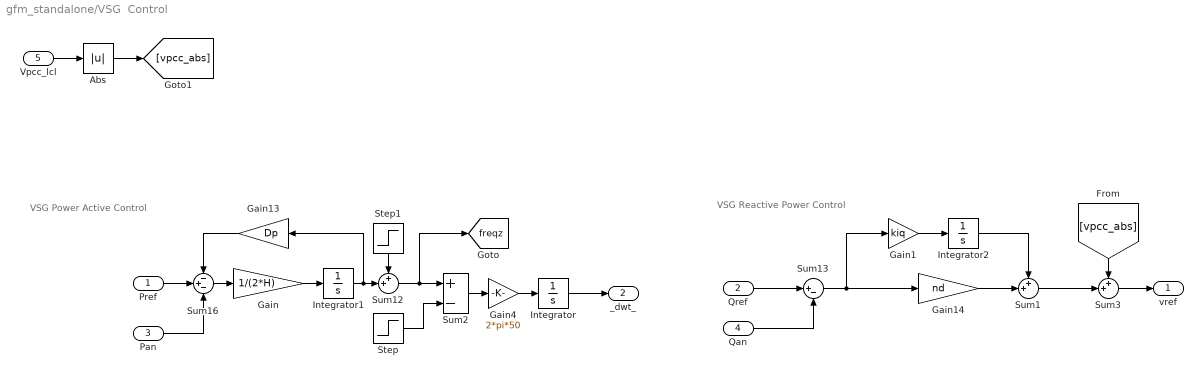
== system gfm_standalone/VSG  Control ==
  note: VSG Reactive Power Control
  note: VSG Power Active Control
  Pref : Inport
  Qref : Inport  Port=2
  Pan : Inport  Port=3
  Qan : Inport  Port=4
  Vpcc_lcl : Inport  Port=5
  Abs : Abs  SaturateOnIntegerOverflow=off
  Gain : Gain  Gain=1/(2*H)
  Gain1 : Gain  Gain=kiq
  Gain13 : Gain  Gain=Dp
  Gain14 : Gain  Gain=nd
  Gain4 : Gain  Gain=2*pi*50
  Integrator : Integrator  InitialCondition=angle(vref_)  ContinuousStateAttributes='psi_theta'
  Integrator1 : Integrator  ContinuousStateAttributes='delta_w'
  Integrator2 : Integrator  ContinuousStateAttributes='qdif'
  Step : Step  Before=1  SampleTime=0
  Step1 : Step  Time=2  Before=1  SampleTime=0
  Sum1 : Sum  Inputs=++|
  Sum12 : Sum  Inputs=++|
  Sum13 : Sum  Inputs=|+-
  Sum16 : Sum  Inputs=-+-
  Sum2 : Sum  Inputs=+-
  Sum3 : Sum  Inputs=++|
  vref : Outport
  _dwt_ : Outport  Port=2
  tag scope: freqz=global
  wires:
  Qref/1 -> Sum13/1
  Sum3/1 -> vref/1
  Qan/1 -> Sum13/2
  Sum13/1 -> Gain1/1, Gain14/1
  Sum2/1 -> Gain4/1
  Gain4/1 -> Integrator/1
  Sum12/1 -> [freqz], Sum2/1
  Integrator/1 -> _dwt_/1
  Sum16/1 -> Gain/1
  Gain/1 -> Integrator1/1
  Integrator1/1 -> Gain13/1, Sum12/2
  Gain13/1 -> Sum16/1
  Gain14/1 -> Sum1/2
  Sum1/1 -> Sum3/2
  Gain1/1 -> Integrator2/1
  Integrator2/1 -> Sum1/1
  Vpcc_lcl/1 -> Abs/1
  Abs/1 -> [vpcc_abs]
  [vpcc_abs] -> Sum3/1
  Step1/1 -> Sum12/1
  Step/1 -> Sum2/2
  Pref/1 -> Sum16/2
  Pan/1 -> Sum16/3

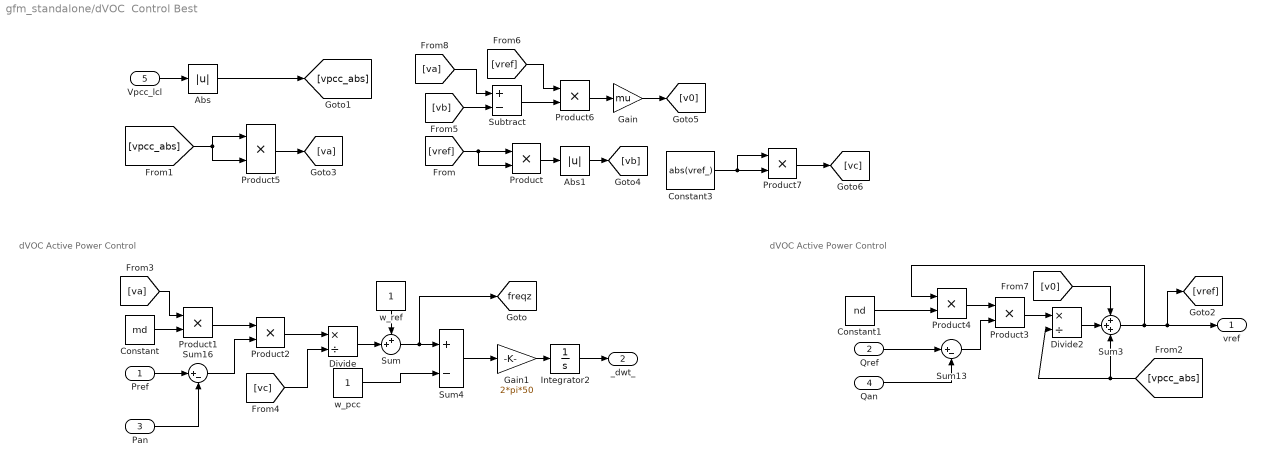
== system gfm_standalone/dVOC  Control Best ==
  note: dVOC Active Power Control
  note: dVOC Active Power Control
  Pref : Inport
  Qref : Inport  Port=2
  Pan : Inport  Port=3
  Qan : Inport  Port=4
  Vpcc_lcl : Inport  Port=5
  Abs : Abs  SaturateOnIntegerOverflow=off
  Abs1 : Abs  SaturateOnIntegerOverflow=off
  Constant : Constant  Value=md
  Constant1 : Constant  Value=nd
  Constant3 : Constant  Value=abs(vref_)
  Divide : Product  Inputs=*/
  Divide2 : Product  Inputs=*/
  Gain : Gain  Gain=mu
  Gain1 : Gain  Gain=2*pi*50
  Integrator2 : Integrator  InitialCondition=angle(vref_)  ContinuousStateAttributes='psi_theta'
  Product{,1..7} (8 alike) : Product
  Subtract : Sum  Inputs=+-
  Sum : Sum  Inputs=++|
  Sum13 : Sum  Inputs=|+-
  Sum16 : Sum  Inputs=|+-
  Sum3 : Sum  Inputs=+++
  Sum4 : Sum  Inputs=+-
  w_pcc : Constant
  w_ref : Constant
  vref : Outport
  _dwt_ : Outport  Port=2
  tag scope: freqz=global
  wires:
  Qref/1 -> Sum13/1
  Qan/1 -> Sum13/2
  Pref/1 -> Sum16/1
  Pan/1 -> Sum16/2
  Vpcc_lcl/1 -> Abs/1
  Constant/1 -> Product1/2
  Sum16/1 -> Product2/2
  Product2/1 -> Divide/1
  Sum4/1 -> Gain1/1
  Gain1/1 -> Integrator2/1
  Integrator2/1 -> _dwt_/1
  Product4/1 -> Product3/1
  Product3/1 -> Divide2/1
  Sum3/1 -> [vref], vref/1, Product4/1
  Product1/1 -> Product2/1
  Sum13/1 -> Product3/2
  [vpcc_abs] -> Product5/1, Product5/2
  Product5/1 -> [va]
  Divide/1 -> Sum/2
  w_ref/1 -> Sum/1
  Sum/1 -> Sum4/1, [freqz]
  w_pcc/1 -> Sum4/2
  Constant1/1 -> Product4/2
  Abs/1 -> [vpcc_abs]
  [vpcc_abs] -> Sum3/3, Divide2/2
  Product/1 -> Abs1/1
  Abs1/1 -> [vb]
  [vref] -> Product/2, Product/1
  Divide2/1 -> Sum3/2
  [vb] -> Subtract/2
  Subtract/1 -> Product6/2
  [vref] -> Product6/1
  Product6/1 -> Gain/1
  Gain/1 -> [v0]
  [va] -> Subtract/1
  [va] -> Product1/1
  [v0] -> Sum3/1
  Product7/1 -> [vc]
  Constant3/1 -> Product7/1, Product7/2
  [vc] -> Divide/2

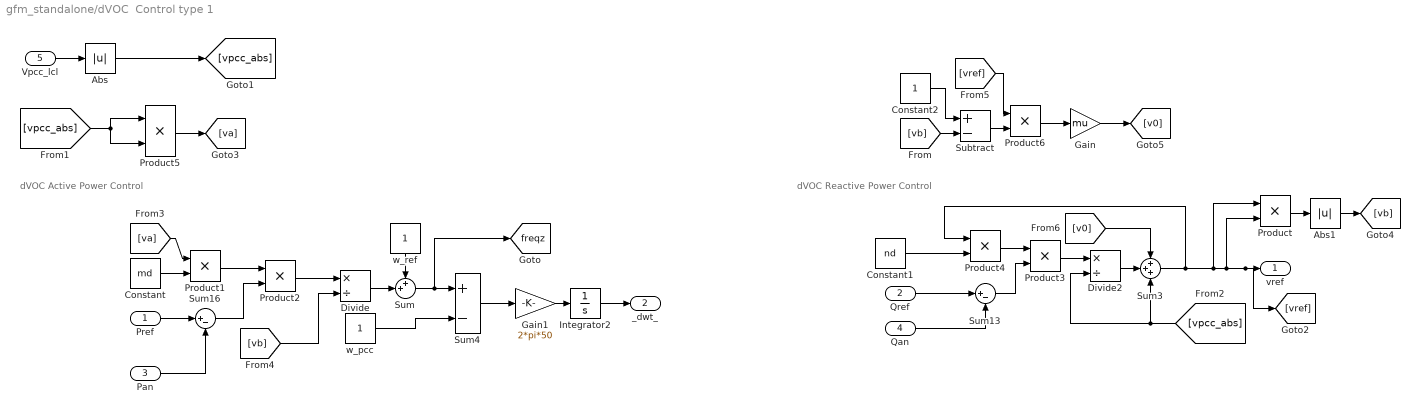
== system gfm_standalone/dVOC  Control type 1 ==
  note: dVOC Active Power Control
  note: dVOC Reactive Power Control
  Pref : Inport
  Qref : Inport  Port=2
  Pan : Inport  Port=3
  Qan : Inport  Port=4
  Vpcc_lcl : Inport  Port=5
  Abs : Abs  SaturateOnIntegerOverflow=off
  Abs1 : Abs  SaturateOnIntegerOverflow=off
  Constant : Constant  Value=md
  Constant1 : Constant  Value=nd
  Constant2 : Constant
  Divide : Product  Inputs=*/
  Divide2 : Product  Inputs=*/
  Gain : Gain  Gain=mu
  Gain1 : Gain  Gain=2*pi*50
  Integrator2 : Integrator  InitialCondition=angle(vref_)
  Product{,1..6} (7 alike) : Product
  Subtract : Sum  Inputs=+-
  Sum : Sum  Inputs=++|
  Sum13 : Sum  Inputs=|+-
  Sum16 : Sum  Inputs=|+-
  Sum3 : Sum  Inputs=+++
  Sum4 : Sum  Inputs=+-
  w_pcc : Constant
  w_ref : Constant
  vref : Outport
  _dwt_ : Outport  Port=2
  tag scope: freqz=global
  wires:
  Qref/1 -> Sum13/1
  Qan/1 -> Sum13/2
  Pref/1 -> Sum16/1
  Pan/1 -> Sum16/2
  Vpcc_lcl/1 -> Abs/1
  Constant/1 -> Product1/2
  Sum16/1 -> Product2/2
  Product2/1 -> Divide/1
  Sum4/1 -> Gain1/1
  Gain1/1 -> Integrator2/1
  Integrator2/1 -> _dwt_/1
  Product4/1 -> Product3/1
  Product3/1 -> Divide2/1
  Sum3/1 -> Product/1, Product/2, [vref], vref/1, Product4/1
  Product1/1 -> Product2/1
  Sum13/1 -> Product3/2
  [vpcc_abs] -> Product5/1, Product5/2
  Product5/1 -> [va]
  Divide/1 -> Sum/2
  w_ref/1 -> Sum/1
  Sum/1 -> Sum4/1, [freqz]
  w_pcc/1 -> Sum4/2
  Constant1/1 -> Product4/2
  Abs/1 -> [vpcc_abs]
  [va] -> Product1/1
  [vb] -> Divide/2
  [vpcc_abs] -> Divide2/2, Sum3/3
  Product/1 -> Abs1/1
  Abs1/1 -> [vb]
  [vb] -> Subtract/2
  Constant2/1 -> Subtract/1
  Subtract/1 -> Product6/2
  [vref] -> Product6/1
  Product6/1 -> Gain/1
  Gain/1 -> [v0]
  Divide2/1 -> Sum3/2
  [v0] -> Sum3/1

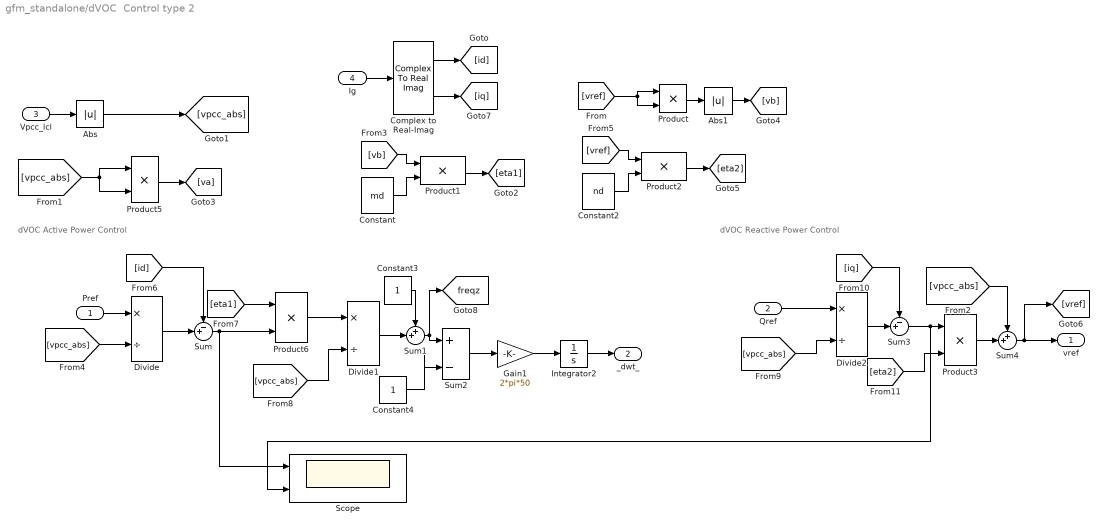
== system gfm_standalone/dVOC  Control type 2 ==
  note: dVOC Active Power Control
  note: dVOC Reactive Power Control
  Pref : Inport
  Qref : Inport  Port=2
  Vpcc_lcl : Inport  Port=3
  Ig : Inport  Port=4
  Abs : Abs  SaturateOnIntegerOverflow=off
  Abs1 : Abs  SaturateOnIntegerOverflow=off
  Complex to Real-Imag : ComplexToRealImag
  Constant : Constant  Value=md
  Constant2 : Constant  Value=nd
  Constant3 : Constant
  Constant4 : Constant
  Divide : Product  Inputs=*/
  Divide1 : Product  Inputs=*/
  Divide2 : Product  Inputs=*/
  Gain1 : Gain  Gain=2*pi*50
  Integrator2 : Integrator  InitialCondition=angle(vref_)
  Product{,1..3,5..6} (6 alike) : Product
  Scope : Scope  NumInputPorts=2
  Sum : Sum  Inputs=-+|
  Sum1 : Sum  Inputs=++|
  Sum2 : Sum  Inputs=+-|
  Sum3 : Sum  Inputs=-+|
  Sum4 : Sum  Inputs=++|
  vref : Outport
  _dwt_ : Outport  Port=2
  tag scope: freqz=global
  wires:
  Qref/1 -> Divide2/1
  Vpcc_lcl/1 -> Abs/1
  Constant/1 -> Product1/2
  Gain1/1 -> Integrator2/1
  Integrator2/1 -> _dwt_/1
  [vpcc_abs] -> Product5/1, Product5/2
  Product5/1 -> [va]
  Abs/1 -> [vpcc_abs]
  [vb] -> Product1/1
  Product/1 -> Abs1/1
  Abs1/1 -> [vb]
  Product1/1 -> [eta1]
  Product2/1 -> [eta2]
  [vref] -> Product2/1
  Constant2/1 -> Product2/2
  [vref] -> Product/1, Product/2
  Ig/1 -> Complex to Real-Imag/1
  Complex to Real-Imag/1 -> [id]
  Complex to Real-Imag/2 -> [iq]
  [vpcc_abs] -> Divide/2
  Pref/1 -> Divide/1
  Divide/1 -> Sum/2
  [id] -> Sum/1
  [eta1] -> Product6/1
  Sum/1 -> Scope/1, Product6/2
  Product6/1 -> Divide1/1
  [vpcc_abs] -> Divide1/2
  Divide1/1 -> Sum1/2
  Sum1/1 -> [freqz], Sum2/1
  Sum2/1 -> Gain1/1
  Constant3/1 -> Sum1/1
  Constant4/1 -> Sum2/2
  [vpcc_abs] -> Divide2/2
  Divide2/1 -> Sum3/2
  [iq] -> Sum3/1
  Sum3/1 -> Scope/2, Product3/1
  [eta2] -> Product3/2
  Product3/1 -> Sum4/2
  [vpcc_abs] -> Sum4/1
  Sum4/1 -> [vref], vref/1

== system gfm_standalone/Converter Control/Subsystem ==
  dq : Inport
  delta_wt : Inport  Port=2
  Complex to Real-Imag1 : ComplexToRealImag
  Divide1 : Product  Inputs=**
  Gain6 : Gain  Gain=-1i
  Math Function : Math  SignedPower=on  RndMeth=Zero
  d : Outport
  q : Outport  Port=2
  wires:
  Math Function/1 -> Divide1/2
  Complex to Real-Imag1/1 -> d/1
  Divide1/1 -> Complex to Real-Imag1/1
  delta_wt/1 -> Gain6/1
  Gain6/1 -> Math Function/1
  dq/1 -> Divide1/1
  Complex to Real-Imag1/2 -> q/1

== system gfm_standalone/Converter Control/Subsystem1 ==
  dq : Inport
  delta_wt : Inport  Port=2
  Complex to Real-Imag1 : ComplexToRealImag
  Divide1 : Product  Inputs=**
  Gain6 : Gain  Gain=-1i
  Math Function : Math  SignedPower=on  RndMeth=Zero
  d : Outport
  q : Outport  Port=2
  wires:
  Math Function/1 -> Divide1/2
  Complex to Real-Imag1/1 -> d/1
  Divide1/1 -> Complex to Real-Imag1/1
  delta_wt/1 -> Gain6/1
  Gain6/1 -> Math Function/1
  dq/1 -> Divide1/1
  Complex to Real-Imag1/2 -> q/1

== system gfm_standalone/Converter Control/Subsystem2 ==
  dq : Inport
  d_wt : Inport  Port=2
  Complex to Real-Imag1 : ComplexToRealImag
  Divide1 : Product  Inputs=**
  Gain6 : Gain  Gain=1i
  Math Function : Math  SignedPower=on  RndMeth=Zero
  d : Outport
  q : Outport  Port=2
  wires:
  Complex to Real-Imag1/1 -> d/1
  Divide1/1 -> Complex to Real-Imag1/1
  d_wt/1 -> Gain6/1
  Gain6/1 -> Math Function/1
  dq/1 -> Divide1/1
  Complex to Real-Imag1/2 -> q/1
  Math Function/1 -> Divide1/2
